simulink model "model2"  (R2021a)
settings: Solver=VariableStepAuto  StartTime=0.0  StopTime=10.0  RelTol=1e-3
libraries: spsACVoltageSourceLib x1, spsThreePhaseSineGeneratorLib x1, spsVariableInductorLib x1, spsVoltageMeasurementLib x1, spspowerguiLib x1
settings Model: Creator=Eng. Ayman  LastModifiedBy=Eng. Ayman

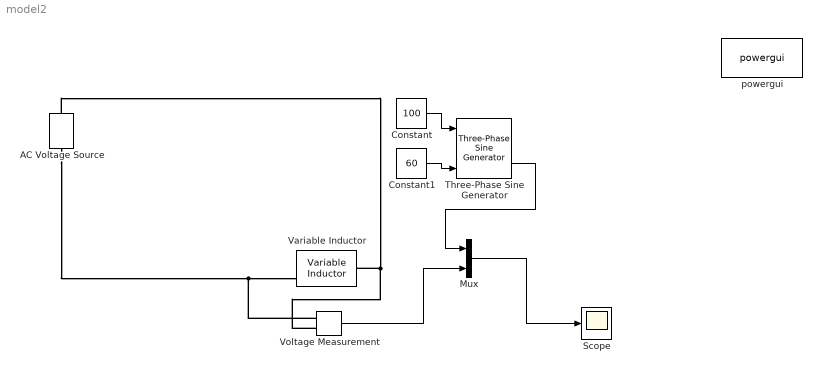
== system model2 ==
  AC Voltage Source : spsACVoltageSourceLib/AC Voltage Source  Amplitude=100  Phase=0  Frequency=60  SampleTime=0  Measurements=None  BusType=swing  Pref=10e3  Qref=0  Qmin=-inf  Qmax=+inf
  Constant : Constant  Value=100
  Constant1 : Constant  Value=60
  Mux : Mux  Inputs=2
  Scope : Scope
  Three-Phase Sine Generator : spsThreePhaseSineGeneratorLib/Three-Phase Sine Generator  Ts=0
      settings: SourceProductBaseCode=PS
  Variable Inductor : spsVariableInductorLib/Variable Inductor  methode=Backward Euler  Labsmin=10  Initialize=off  iL0=0  L0=1e-3  Vl0=0
      settings: SourceProductBaseCode=PS
  Voltage Measurement : spsVoltageMeasurementLib/Voltage Measurement  PhasorSimulation=off  OutputType=Complex  PSBequivalent=0
  powergui : spspowerguiLib/powergui  Priority=1  SimulationMode=Continuous  SampleTime=50e-6  frequency=60  Iterations=50  frequencyindice=60  Pbase=100e6  ErrMax=1e-4  UnitsV=kV  UnitsW=MW  buscounter=0  FunctionMessages=off  echomessages=off  EnableUseOfTLC=off  CurrentSourceSwitches=off  DisableSnubberDevices=off  DisableRonSwitches=off  DisableVfSwitches=off  DisplayEquations=off  AutomaticDiscreteSolvers=off  SolverType=Tustin/Backward Euler (TBE)  Interpol=off  ExternalGateDelay=off  methode=off  Ts=100  x0status=blocks  SPID=on  SwTol=0  HookPort=off  NonlinearTolerance=1e-4  nMaxIteration=100  ContinueOnMaxIteration=off  RestoreLinks=warning  ResistiveCurrentMeasurement=off  Frange=[0:2:500]  Ylog=off  Xlog=on  ShowGrid=off  save=off  variable=ZData  structure=0  ZoomFFT=off  StartTime=0.0  cycles=1  DisplayStyle=1  fundamental=60  FreqAxis=off  MaxFrequency=1000  frequencyindicesteady=1  RmsSteady=1  display=off
  wires:
  Voltage Measurement/1 -> Mux/2
  Three-Phase Sine Generator/2 -> Mux/1
  Constant1/1 -> Three-Phase Sine Generator/3
  Constant/1 -> Three-Phase Sine Generator/1
  Mux/1 -> Scope/1
  connections:
  AC Voltage Source/LConn1 -- Voltage Measurement/LConn1 -- Variable Inductor/LConn1
  AC Voltage Source/RConn1 -- Voltage Measurement/LConn2 -- Variable Inductor/RConn1
